simulink model "sl_subsys_fcncall10"  (Simulink 7.6)
settings: Solver=FixedStepDiscrete  StartTime=0.0  StopTime=10.0  FixedStep=1  RelTol=1e-3
Description:
  | Nested function-call
  | 
  | The Chart below is a function-call initiator that executes the function, [d1,d2]=f().
  | The function f, in turn, executes the function g. After invoking f and g, the Chart uses the values d1 and d2 computed by f and g.
settings Model: Creator=The MathWorks Inc.  CovMetricSettings=d  ExtModeAutoUpdateStatusClock=off
settings OptimizationCC: BlockReduction=off  BooleanDataType=off  InlineInvariantSignals=on  InitFltsAndDblsToZero=on
settings DebuggingCC: SaveWithParameterizedLinksMsg=none  SignalResolutionControl=TryResolveAllWithWarning  SolverPrmCheckMsg=none  MultiTaskDSMMsg=warning  MultiTaskCondExecSysMsg=none
settings HardwareCC: TargetUnknown=on
settings SFSimCC: SimParseCustomCode=off
settings RTWCC: IncludeERTFirstTime=on
settings CodeAppCC: CustomSymbolStrFcn=$F$N$M
settings GRTTargetCC: TargetFcnLib=ansi_tfl_tmw.mat

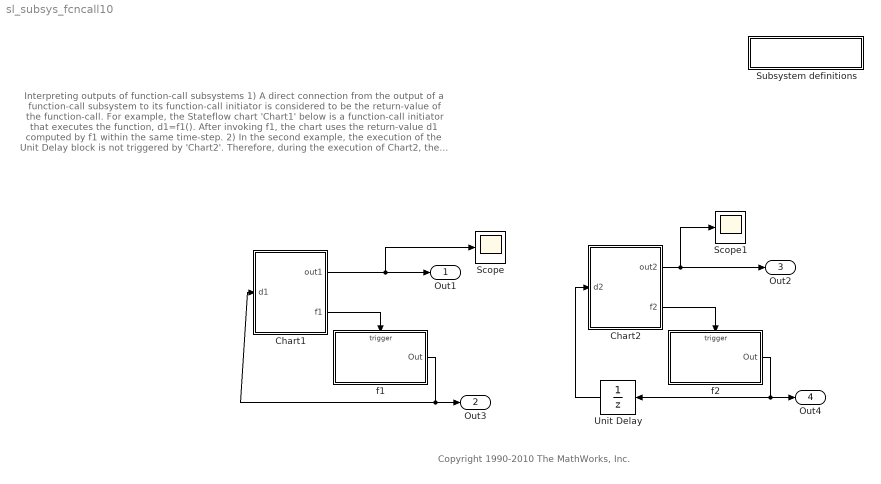
== system sl_subsys_fcncall10 ==
  note: Interpreting outputs of function-call subsystems
      |
      | 1) A direct connection from the output of a function-call subsystem to its
      | function-call initiator is considered to be the return-value of the function-call.
      | For example, the Stateflow chart 'Chart1' below is a function-call initiator
      | that executes the function, d1=f1().  After invoking f1, the chart uses the
      | return-value d1 computed by f1 within the same time-step.
      |
      | 2) In the second example, the execution of the Unit Delay block is not triggered
      | by 'Chart2'. Therefore, during the execution of Chart2, the signal d2 maintains
      | its value from the previous time-step at which the Unit Delay was invoked.
      |
      | 3) See sl_subsys_fcncallerr1.
  note: Copyright 1990-2010 The MathWorks, Inc.
  " Subsystem definitions" : Subsystem
      settings: OpenFcn=helpview([matlabroot,'/toolbox/simulink/simdemos/simfeatures/html/sl_subsys_definitions.html']);
      mask Display: disp('Subsystem\ndefinitions')
  Chart1 : Stateflow chart  TreatAsAtomicUnit=on
  Chart2 : Stateflow chart  TreatAsAtomicUnit=on
  Scope : Scope
  Scope1 : Scope
  Unit Delay : UnitDelay
  f1 : Subsystem  TreatAsAtomicUnit=on
  f2 : Subsystem  TreatAsAtomicUnit=on
  Out1 : Outport
  Out3 : Outport  Port=2
  Out2 : Outport  Port=3
  Out4 : Outport  Port=4
  wires:
  Chart1/2(f1) -> f1/Trigger
  f1/1(Out) -> Out3/1, Chart1/1(d1)
  Chart1/1(out1) -> Out1/1, Scope/1
  Chart2/2(f2) -> f2/Trigger
  f2/1(Out) -> Out4/1, Unit Delay/1
  Chart2/1(out2) -> Out2/1, Scope1/1
  Unit Delay/1 -> Chart2/1(d2)

== system sl_subsys_fcncall10/ Subsystem definitions ==

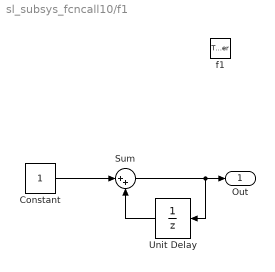
== system sl_subsys_fcncall10/f1 ==
  f1 : TriggerPort  TriggerType=function-call
  Constant : Constant
  Sum : Sum  Inputs=|++  SaturateOnIntegerOverflow=on  InputSameDT=on  OutDataTypeStr=Inherit: Same as first input
  Unit Delay : UnitDelay  SampleTime=-1
  Out : Outport
  wires:
  Constant/1 -> Sum/1
  Unit Delay/1 -> Sum/2
  Sum/1 -> Out/1, Unit Delay/1

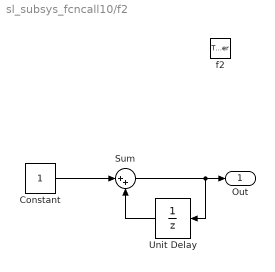
== system sl_subsys_fcncall10/f2 ==
  f2 : TriggerPort  TriggerType=function-call
  Constant : Constant
  Sum : Sum  Inputs=|++  SaturateOnIntegerOverflow=on  InputSameDT=on  OutDataTypeStr=Inherit: Same as first input
  Unit Delay : UnitDelay  SampleTime=-1
  Out : Outport
  wires:
  Sum/1 -> Unit Delay/1, Out/1
  Unit Delay/1 -> Sum/2
  Constant/1 -> Sum/1

== stateflow chart Chart1 ==
  state one/
    entry:f1;out1=d1;
  state two/
    entry: f1;out1=-d1;
  one -> two
  two -> one
  (default) -> one
  data: d1 input double; out1 output double
  events: f1 output FUNCTION_CALL_EVENT

== stateflow chart Chart2 ==
  state one/
    entry:f2;out2=d2;
  state two/
    entry: f2;out2=-d2;
  one -> two
  two -> one
  (default) -> one
  data: d2 input double; out2 output double
  events: f2 output FUNCTION_CALL_EVENT
